simulink model "cartpole_discrete"  (R2019b)
settings: Solver=FixedStepAuto  StartTime=0.0  StopTime=10000  MaxStep=1e-2  RelTol=1e-3
model workspace (MATLAB code in the model file):
  | mCart = 1;
  | mPend = 1;
  | g = 9.81;
  | L = 0.5;
  | theta0 = 0;
  | Kd = 10;
values from neighbouring files (symbols this model uses):
  initialPos = 0    [bonsaiAssess.m]    (also in bonsaiAssessData.m)
libraries: bonsai_library x1
settings Model: Creator=The MathWorks, Inc.  LastModifiedBy=evankramer
settings SolverCC: AlgebraicLoopSolver=LineSearch
settings DataIOCC: LimitDataPoints=on  SaveFormat=Array  ReturnWorkspaceOutputs=off  OutputOption=SpecifiedOutputTimes  OutputTimes=0:1/30:12
settings OptimizationCC: LifeSpan=inf
settings DebuggingCC: AlgebraicLoopMsg=error  UnderspecifiedInitializationDetection=Classic  MergeDetectMultiDrivingBlocksExec=none  SolverPrmCheckMsg=warning  StateNameClashWarn=warning  SFUnexpectedBacktrackingDiag=warning  SFNoUnconditionalDefaultTransitionDiag=warning  SFExecutionAtInitializationDiag=none  ArithmeticOperatorsInVariantConditions=warning
settings HardwareCC: ProdBitPerPointer=32  ProdBitPerSizeT=32  ProdBitPerPtrDiffT=32  ProdLargestAtomicFloat=None  ProdIntDivRoundTo=Undefined  ProdEndianess=Unspecified  ProdWordSize=32  ProdHWDeviceType=32-bit Generic
settings ModelReferenceCC: PropagateSignalLabelsOutOfModel=off
settings SFSimCC: SimUseLocalCustomCode=off  CustomCodeUndefinedFunction=UseInterfaceOnly
settings RTWCC: RTWUseLocalCustomCode=off
settings CodeAppCC: StateflowObjectComments=on
settings GRTTargetCC: TargetLangStandard=C89/C90 (ANSI)
settings ConfigComp: CovMetricSettings=dw  CovHtmlReporting=on  CovSaveCumulativeToWorkspaceVar=on  CovSaveSingleToWorkspaceVar=on  CovExternalEMLEnable=off  CovSFcnEnable=off
settings SimscapeCC: SimscapeNormalizeSystem=off
settings ConfigurationSet: Description=SimMechanics 2G
settings ExplorerConfigSet: InternalSimMechanicsExplorerSettings="<ExplorerConfiguration><canonicalview>default</canonicalview><TilePanel><TileInfo><Tiles Columns=\"1\" Count=\"1\" Rows=\"1\"><Column Left=\"2\" Weight=\"1\"/><Column Left=\"591\"/><Row Top=\"2\" Weight=\"1\"/><Row Top=\"389\"/><Tile Height=\"1\" Width=\"1\" X=\"0\" Y=\"0\"/></Tiles></TileInfo><SceneInfo><SceneViewer><BGColor><R>0.60000002384185791</R><G>0.60000002384185791</G><B>0.60000002384185791</B></BGColor><Camera><Position><X>0.64243946887929204</X><Y>-49.663614699976236</Y><Z>0.22319801622928798</Z></Position><Center><X>0.64243946887929204</X><Y>0</Y><Z>0.22319801622928798</Z></Center><Up><X>0</X><Y>-0</Y><Z>1</Z></Up><Left>-0.88124258449330872</Left><Right>0.88124258449330872</Right><Bottom>-0.30475961919215644</Bottom><Top>0.30475961919215644</Top></Camera></SceneViewer></SceneInfo></TilePanel></ExplorerConfiguration>"

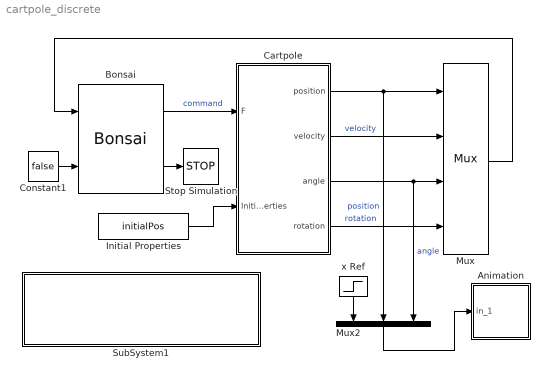
== system cartpole_discrete ==
  Animation : Subsystem  mask(Pendulum plot){RefBlock=x Ref}
      mask prompts: RefBlock "Cart Reference Signal Block Name:"
      mask help: Pendulum plot
      mask Help: Pendulum animation function using Handle graphics.
      mask Display: plot([-10 10],[0 0],[-2 -2 2 2],[0 1 1 0],[0 3],[1 5])
  Bonsai : bonsai_library/Bonsai  sampleTime=[0.1, 0]
      settings: SourceProductName=Bonsai Toolbox
  Cartpole : Subsystem  TreatAsAtomicUnit=on
  Constant1 : Constant  Value=false
  Initial Properties : Constant  Value=initialPos  SampleTime=0.1
  Mux : Mux
      settings: DisplayOption=signals
  Mux2 : Mux  Inputs=3
  Stop Simulation : Stop
  SubSystem1 : Subsystem
      settings: OpenFcn=web('https://preview.bons.ai');
      mask Display:
      | disp(['{', ...
      |     '\fontsize{9}', ...
      |     'After starting bonsaiTrain, double-click here to\newline', ...
      |     'open https://preview.bons.ai and select or create\newline', ...
      |     'a brain to begin training. Hit "Train" and select\newline', ...
      |     'simulator "Simulink Cartpole" to connect this model.', ...
      |     '}'], 'texmode','on');
  x Ref : Step  After=10  SampleTime=0
  wires:
  Mux2/1 -> Animation/1(in_1)
  x Ref/1 -> Mux2/1
  Bonsai/1 -> Cartpole/1(F)  "command"
  Cartpole/1(position) -> Mux/1, Mux2/2  "position"
  Cartpole/2(velocity) -> Mux/2  "velocity"
  Cartpole/4(rotation) -> Mux/4  "rotation"
  Cartpole/3(angle) -> Mux/3, Mux2/3  "angle"
  Mux/1 -> Bonsai/1
  Constant1/1 -> Bonsai/2
  Bonsai/2 -> Stop Simulation/1
  Initial Properties/1 -> Cartpole/2(Initial Properties)

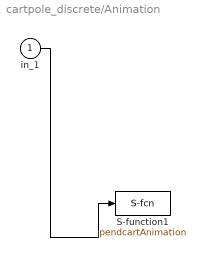
== system cartpole_discrete/Animation ==
  in_1 : Inport
  S-function1 : S-Function  FunctionName=pendcartAnimation  Parameters=RefBlock  SFunctionDeploymentMode=off  EnableBusSupport=off
      settings: DeleteFcn=pendcartAnimation([],[],[],'DeleteBlock');
  wires:
  in_1/1 -> S-function1/1

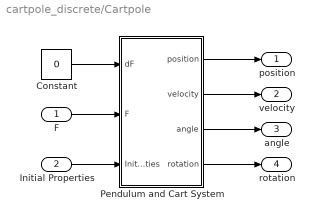
== system cartpole_discrete/Cartpole ==
  F : Inport
  Initial Properties : Inport  Port=2
  Constant : Constant  Value=0
  Pendulum and Cart System : Subsystem  mask{mCartPara=1, mPendPara=0.1, gPara=9.81, LPara=1, KdPara=0}
      mask prompts: mCartPara "Mass of Cart"; mPendPara "Mass of Pendulum"; gPara "Gravity"; LPara "Length of Pendulum"; KdPara "Friction coefficient of Cart"
      mask help: Pendulum and Cart System
      mask init:
      | mCart = str2double(get_param(gcb,'mCartPara'));
      | mPend = str2double(get_param(gcb,'mPendPara'));
      | g = str2double(get_param(gcb,'gPara'));
      | L = str2double(get_param(gcb,'LPara'));
      | Kd = str2double(get_param(gcb,'KdPara'));
  position : Outport  VectorParamsAs1DForOutWhenUnconnected=off
  velocity : Outport  Port=2  VectorParamsAs1DForOutWhenUnconnected=off
  angle : Outport  Port=3  VectorParamsAs1DForOutWhenUnconnected=off
  rotation : Outport  Port=4  VectorParamsAs1DForOutWhenUnconnected=off
  wires:
  Pendulum and Cart System/4(rotation) -> rotation/1
  Pendulum and Cart System/3(angle) -> angle/1
  F/1 -> Pendulum and Cart System/2(F)
  Pendulum and Cart System/2(velocity) -> velocity/1
  Pendulum and Cart System/1(position) -> position/1
  Constant/1 -> Pendulum and Cart System/1(dF)
  Initial Properties/1 -> Pendulum and Cart System/3(Initial Properties)

== system cartpole_discrete/SubSystem1 ==

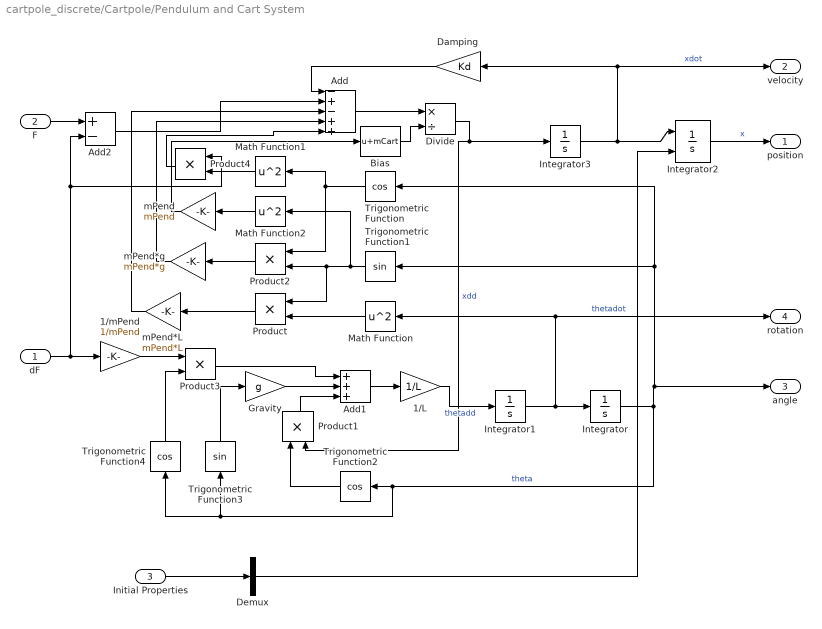
== system cartpole_discrete/Cartpole/Pendulum and Cart System ==
  dF : Inport
  F : Inport  Port=2
  Initial Properties : Inport  Port=3
  1/L : Gain  Gain=1/L
  1/mPend : Gain  Gain=1/mPend
  Add : Sum  Inputs=-+-++
  Add1 : Sum  Inputs=+++
  Add2 : Sum  Inputs=+-
  Bias : Bias  Bias=mCart
  Damping : Gain  Gain=Kd
  Demux : Demux  Outputs=1
  Divide : Product  Inputs=*/
  Gravity : Gain  Gain=g
  Integrator : Integrator
  Integrator1 : Integrator
  Integrator2 : Integrator  InitialConditionSource=external  InitialCondition=initialPos
  Integrator3 : Integrator
  Math Function : Math  Operator=square  SaturateOnIntegerOverflow=on
  Math Function1 : Math  Operator=square  SaturateOnIntegerOverflow=on
  Math Function2 : Math  Operator=square  SaturateOnIntegerOverflow=on
  Product{,1..4} (5 alike) : Product
  Trigonometric Function : Trigonometry  Operator=cos
  Trigonometric Function1 : Trigonometry
  Trigonometric Function2 : Trigonometry  Operator=cos
  Trigonometric Function3 : Trigonometry
  Trigonometric Function4 : Trigonometry  Operator=cos
  mPend : Gain  Gain=mPend
  mPend*L : Gain  Gain=mPend*L
  mPend*g : Gain  Gain=mPend*g
  position : Outport  VectorParamsAs1DForOutWhenUnconnected=off
  velocity : Outport  Port=2  VectorParamsAs1DForOutWhenUnconnected=off
  angle : Outport  Port=3  VectorParamsAs1DForOutWhenUnconnected=off
  rotation : Outport  Port=4  VectorParamsAs1DForOutWhenUnconnected=off
  wires:
  mPend/1 -> Bias/1
  Bias/1 -> Divide/2
  Math Function2/1 -> mPend/1
  Product4/1 -> Add/5
  Math Function1/1 -> Product4/2
  mPend*g/1 -> Add/4
  Product1/1 -> Add1/3
  Math Function/1 -> Product/2
  1/L/1 -> Integrator1/1  "thetadd"
  dF/1 -> 1/mPend/1, Product4/1, Add2/2
  1/mPend/1 -> Product3/1
  Trigonometric Function4/1 -> Product3/2
  Damping/1 -> Add/1
  F/1 -> Add2/1
  Trigonometric Function3/1 -> Gravity/1
  Gravity/1 -> Add1/2
  Trigonometric Function/1 -> Math Function1/1, Product2/1
  Integrator1/1 -> Integrator/1, Math Function/1, rotation/1  "thetadot"
  Integrator/1 -> Trigonometric Function/1, Trigonometric Function1/1, angle/1, Trigonometric Function2/1, Trigonometric Function3/1, Trigonometric Function4/1  "theta"
  Product3/1 -> Add1/1
  Add/1 -> Divide/1
  Divide/1 -> Integrator3/1, Product1/2  "xdd"
  Trigonometric Function2/1 -> Product1/1
  Trigonometric Function1/1 -> Math Function2/1, Product/1, Product2/2
  Integrator2/1 -> position/1  "x"
  Integrator3/1 -> Damping/1, velocity/1, Integrator2/1  "xdot"
  Product2/1 -> mPend*g/1
  Add1/1 -> 1/L/1
  Add2/1 -> Add/2
  mPend*L/1 -> Add/3
  Product/1 -> mPend*L/1
  Initial Properties/1 -> Demux/1
  Demux/1 -> Integrator2/2
